simulink model "vector_susp_ctrl_canoe"  (R2012b)
settings: Solver=ode3  StartTime=0.0  StopTime=10.0  FixedStep=T  RelTol=1e-3
PreLoadFcn:
  | init_parameters;
libraries: canoelib x27
settings Model: Creator=vismso  LastModifiedBy=vikafla
settings DataIOCC: SignalLoggingSaveFormat=ModelDataLogs  SaveOutput=off  SignalLogging=off  SaveTime=off
settings OptimizationCC: InlineParams=on  UseIntDivNetSlope=on  InlineInvariantSignals=on  SimCompilerOptimization=On
settings DebuggingCC: FcnCallInpInsideContextMsg=UseLocalSettings  StrictBusMsg=Warning
settings RTWCC: SystemTargetFile=cn.tlc  TemplateMakefile=cn_msdll.tmf  Description=Vector CANoe Real-Time Target DLL (Visual C/C++ Project Makefile)  ProcessScript=cn_make_rtw_hook
settings CodeAppCC: MaxIdLength=128
settings STFCustomTargetCC: CodeReplacementLibrary=ANSI_C  GeneratePreprocessorConditionals=Disable all  MatFileLogging=on  SystemTargetFile=cn.tlc
settings GRTTargetCC: ParMdlRefBuildCompliant=off  CompOptLevelCompliant=off  ConcurrentExecutionCompliant=off  CombineOutputUpdateFcns=off  GRTInterface=on  ExtModeMexFile=noextcomm  RTWCAPISignals=on  RTWCAPIParams=on

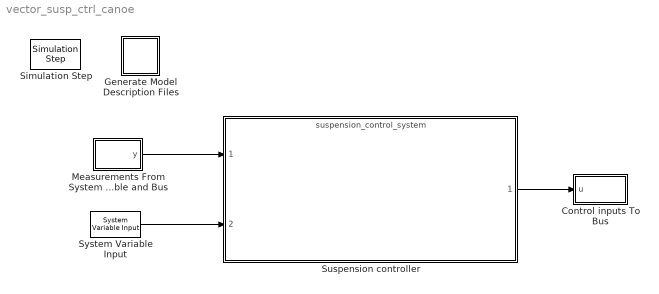
== system vector_susp_ctrl_canoe ==
  Control inputs To Bus : Subsystem
  Generate Model Description Files : Subsystem  mask{enable=off}
      mask prompts: enable "Enabled?"
      mask init:
      | x=1; y=1;
      | if( enable )
      |     x=[0 1 2];
      |     y=[1 0 2];
      | else
      |     x=[0 1 2 1 2 0];
      |     y=[0 1 2 1 0 2];
      | end
      settings: OpenFcn=callback_rtwoptionset;
      mask Display: plot(x,y)
  Measurements From System Variable and Bus : Subsystem
  Simulation Step : canoelib/CANoe I//O/Simulation Step  mode=Synchronized
      settings: AttributesFormatString=%<mode>
  Suspension controller : ModelReference  ModelNameDialog=suspension_control_system  SimulationMode=Normal  ModelReferenceVersion=1.1903  CopyOfModelName=suspension_control_system  DefaultDataLogging=off
  System Variable Input : canoelib/CANoe I//O/System Variable Input  nsName=ModelStimuli  sysVarName=Susp_Ctrl_Select  arrayIndex=-1  editSampleTime=0  rawValue=Default  dataType=Default  dataTypeDB=unknown  hasEncoding=off  dataTypeCANoe=Get from CANoe
      settings: AttributesFormatString=%<nsName>::%<sysVarName>
  wires:
  Suspension controller/1 -> Control inputs To Bus/1(u)
  System Variable Input/1 -> Suspension controller/2
  Measurements From System Variable and Bus/1(y) -> Suspension controller/1

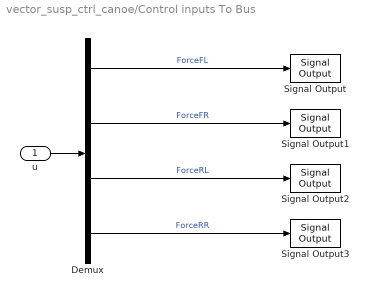
== system vector_susp_ctrl_canoe/Control inputs To Bus ==
  u : Inport
  Demux : Demux
  Signal Output : canoelib/CANoe I//O/Signal Output  SystemSampleTime=-1  dbName=""  nodeName=""  msgName=""  sigName=Susp_Ctrl_DesiredForce_FL  rawValue=off
      settings: AttributesFormatString=%<sigName>
  Signal Output1 : canoelib/CANoe I//O/Signal Output  SystemSampleTime=-1  dbName=""  nodeName=""  msgName=""  sigName=Susp_Ctrl_DesiredForce_FR  rawValue=off
      settings: AttributesFormatString=%<sigName>
  Signal Output2 : canoelib/CANoe I//O/Signal Output  SystemSampleTime=-1  dbName=""  nodeName=""  msgName=""  sigName=Susp_Ctrl_DesiredForce_RL  rawValue=off
      settings: AttributesFormatString=%<sigName>
  Signal Output3 : canoelib/CANoe I//O/Signal Output  SystemSampleTime=-1  dbName=""  nodeName=""  msgName=""  sigName=Susp_Ctrl_DesiredForce_RR  rawValue=off
      settings: AttributesFormatString=%<sigName>
  wires:
  Demux/1 -> Signal Output/1  "ForceFL"
  Demux/2 -> Signal Output1/1  "ForceFR"
  Demux/3 -> Signal Output2/1  "ForceRL"
  Demux/4 -> Signal Output3/1  "ForceRR"
  u/1 -> Demux/1

== system vector_susp_ctrl_canoe/Generate Model Description Files ==

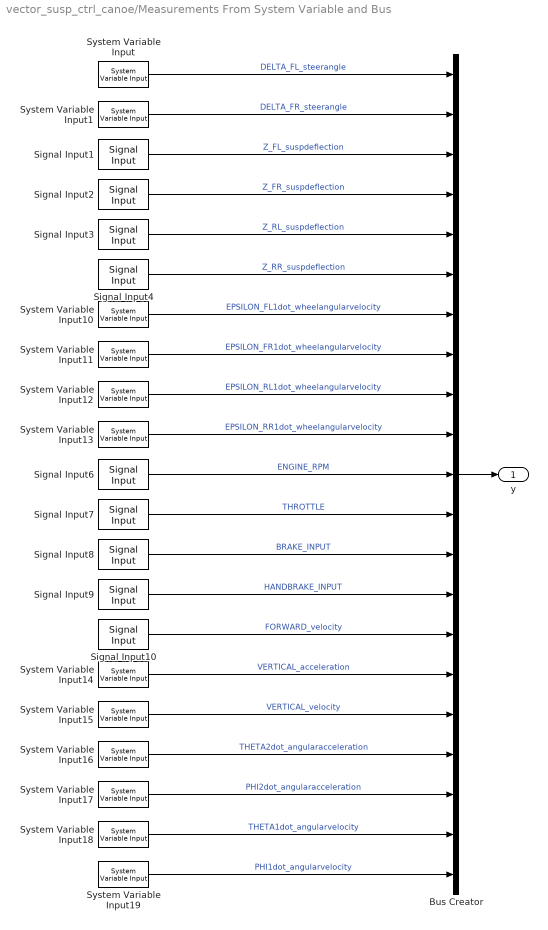
== system vector_susp_ctrl_canoe/Measurements From System Variable and Bus ==
  Bus Creator : BusCreator  Inputs=21  OutDataTypeStr=Bus: Bus_Measurements
  Signal Input1 : canoelib/CANoe I//O/Signal Input  SystemSampleTime=-1  dbName=""  nodeName=""  msgName=""  sigName=Susp_Ctrl_SuspDefl_FL  editSampleTime=0  rawValue=off
      settings: AttributesFormatString=%<sigName>
  Signal Input10 : canoelib/CANoe I//O/Signal Input  SystemSampleTime=-1  dbName=""  nodeName=""  msgName=""  sigName=Vehicle_ForwardSpeed  editSampleTime=0  rawValue=off
      settings: AttributesFormatString=%<sigName>
  Signal Input2 : canoelib/CANoe I//O/Signal Input  SystemSampleTime=-1  dbName=""  nodeName=""  msgName=""  sigName=Susp_Ctrl_SuspDefl_FR  editSampleTime=0  rawValue=off
      settings: AttributesFormatString=%<sigName>
  Signal Input3 : canoelib/CANoe I//O/Signal Input  SystemSampleTime=-1  dbName=""  nodeName=""  msgName=""  sigName=Susp_Ctrl_SuspDefl_RL  editSampleTime=0  rawValue=off
      settings: AttributesFormatString=%<sigName>
  Signal Input4 : canoelib/CANoe I//O/Signal Input  SystemSampleTime=-1  dbName=""  nodeName=""  msgName=""  sigName=Susp_Ctrl_SuspDefl_RR  editSampleTime=0  rawValue=off
      settings: AttributesFormatString=%<sigName>
  Signal Input6 : canoelib/CANoe I//O/Signal Input  SystemSampleTime=-1  dbName=""  nodeName=""  msgName=""  sigName=Eng_RPM  editSampleTime=0  rawValue=off
      settings: AttributesFormatString=%<sigName>
  Signal Input7 : canoelib/CANoe I//O/Signal Input  SystemSampleTime=-1  dbName=""  nodeName=""  msgName=""  sigName=Eng_Throttle  editSampleTime=0  rawValue=off
      settings: AttributesFormatString=%<sigName>
  Signal Input8 : canoelib/CANoe I//O/Signal Input  SystemSampleTime=-1  dbName=""  nodeName=""  msgName=""  sigName=Vehicle_BrakePedal  editSampleTime=0  rawValue=off
      settings: AttributesFormatString=%<sigName>
  Signal Input9 : canoelib/CANoe I//O/Signal Input  SystemSampleTime=-1  dbName=""  nodeName=""  msgName=""  sigName=Vehicle_Handbrake  editSampleTime=0  rawValue=off
      settings: AttributesFormatString=%<sigName>
  System Variable Input : canoelib/CANoe I//O/System Variable Input  SystemSampleTime=-1  nsName=ModelLocalMeasurements  sysVarName=SteerAngleFL  arrayIndex=-1  editSampleTime=0
      settings: AttributesFormatString=%<nsName>::%<sysVarName>
  System Variable Input1 : canoelib/CANoe I//O/System Variable Input  SystemSampleTime=-1  nsName=ModelLocalMeasurements  sysVarName=SteerAngleFR  arrayIndex=-1  editSampleTime=0
      settings: AttributesFormatString=%<nsName>::%<sysVarName>
  System Variable Input10 : canoelib/CANoe I//O/System Variable Input  SystemSampleTime=-1  nsName=ModelLocalMeasurements  sysVarName=WheelSpeedFL  arrayIndex=-1  editSampleTime=0
      settings: AttributesFormatString=%<nsName>::%<sysVarName>
  System Variable Input11 : canoelib/CANoe I//O/System Variable Input  SystemSampleTime=-1  nsName=ModelLocalMeasurements  sysVarName=WheelSpeedFR  arrayIndex=-1  editSampleTime=0
      settings: AttributesFormatString=%<nsName>::%<sysVarName>
  System Variable Input12 : canoelib/CANoe I//O/System Variable Input  SystemSampleTime=-1  nsName=ModelLocalMeasurements  sysVarName=WheelSpeedRL  arrayIndex=-1  editSampleTime=0
      settings: AttributesFormatString=%<nsName>::%<sysVarName>
  System Variable Input13 : canoelib/CANoe I//O/System Variable Input  SystemSampleTime=-1  nsName=ModelLocalMeasurements  sysVarName=WheelSpeedRR  arrayIndex=-1  editSampleTime=0
      settings: AttributesFormatString=%<nsName>::%<sysVarName>
  System Variable Input14 : canoelib/CANoe I//O/System Variable Input  SystemSampleTime=-1  nsName=ModelLocalMeasurements  sysVarName=BodyVerticalAcc  arrayIndex=-1  editSampleTime=0
      settings: AttributesFormatString=%<nsName>::%<sysVarName>
  System Variable Input15 : canoelib/CANoe I//O/System Variable Input  SystemSampleTime=-1  nsName=ModelLocalMeasurements  sysVarName=BodyVerticalVel  arrayIndex=-1  editSampleTime=0
      settings: AttributesFormatString=%<nsName>::%<sysVarName>
  System Variable Input16 : canoelib/CANoe I//O/System Variable Input  SystemSampleTime=-1  nsName=ModelLocalMeasurements  sysVarName=BodyPitchAcc  arrayIndex=-1  editSampleTime=0
      settings: AttributesFormatString=%<nsName>::%<sysVarName>
  System Variable Input17 : canoelib/CANoe I//O/System Variable Input  SystemSampleTime=-1  nsName=ModelLocalMeasurements  sysVarName=BodyRollAcc  arrayIndex=-1  editSampleTime=0
      settings: AttributesFormatString=%<nsName>::%<sysVarName>
  System Variable Input18 : canoelib/CANoe I//O/System Variable Input  SystemSampleTime=-1  nsName=ModelLocalMeasurements  sysVarName=BodyPitchVel  arrayIndex=-1  editSampleTime=0
      settings: AttributesFormatString=%<nsName>::%<sysVarName>
  System Variable Input19 : canoelib/CANoe I//O/System Variable Input  SystemSampleTime=-1  nsName=ModelLocalMeasurements  sysVarName=BodyRollVel  arrayIndex=-1  editSampleTime=0
      settings: AttributesFormatString=%<nsName>::%<sysVarName>
  y : Outport  OutDataTypeStr=Bus: Bus_Measurements
  wires:
  Bus Creator/1 -> y/1
  System Variable Input/1 -> Bus Creator/1  "DELTA_FL_steerangle"
  System Variable Input1/1 -> Bus Creator/2  "DELTA_FR_steerangle"
  Signal Input1/1 -> Bus Creator/3  "Z_FL_suspdeflection"
  Signal Input2/1 -> Bus Creator/4  "Z_FR_suspdeflection"
  Signal Input3/1 -> Bus Creator/5  "Z_RL_suspdeflection"
  Signal Input4/1 -> Bus Creator/6  "Z_RR_suspdeflection"
  System Variable Input10/1 -> Bus Creator/7  "EPSILON_FL1dot_wheelangularvelocity"
  System Variable Input11/1 -> Bus Creator/8  "EPSILON_FR1dot_wheelangularvelocity"
  System Variable Input12/1 -> Bus Creator/9  "EPSILON_RL1dot_wheelangularvelocity"
  System Variable Input13/1 -> Bus Creator/10  "EPSILON_RR1dot_wheelangularvelocity"
  Signal Input6/1 -> Bus Creator/11  "ENGINE_RPM"
  Signal Input7/1 -> Bus Creator/12  "THROTTLE"
  Signal Input8/1 -> Bus Creator/13  "BRAKE_INPUT"
  Signal Input9/1 -> Bus Creator/14  "HANDBRAKE_INPUT"
  Signal Input10/1 -> Bus Creator/15  "FORWARD_velocity"
  System Variable Input14/1 -> Bus Creator/16  "VERTICAL_acceleration"
  System Variable Input15/1 -> Bus Creator/17  "VERTICAL_velocity"
  System Variable Input16/1 -> Bus Creator/18  "THETA2dot_angularacceleration"
  System Variable Input17/1 -> Bus Creator/19  "PHI2dot_angularacceleration"
  System Variable Input18/1 -> Bus Creator/20  "THETA1dot_angularvelocity"
  System Variable Input19/1 -> Bus Creator/21  "PHI1dot_angularvelocity"
